simulink model "is95fwdchendtoend2"  (Simulink 4.00)
settings: Solver=VariableStepDiscrete  SolverMode=SingleTasking  StartTime=0.0  StopTime=600  RelTol=1e-3  AbsTol=1e-6
undefined symbols (not defined in the file): Fs
libraries: cdmalibv1p1 x14, cdmaprivate x9, dspsnks3 x3, dspbuff3 x3, commutil2 x3, commsink2 x2, dspsigattribs x2, commchan2 x2
settings Model: RequirementInfo=9  CovMetricSettings=d  Creator=pc  LastModifiedBy=akansal  SaveTime=off  SaveOutput=off  LimitDataPoints=off  ExtModeTrigMode=oneshot  ExtModeArmWhenConnect=off  BlockReductionOpt=off

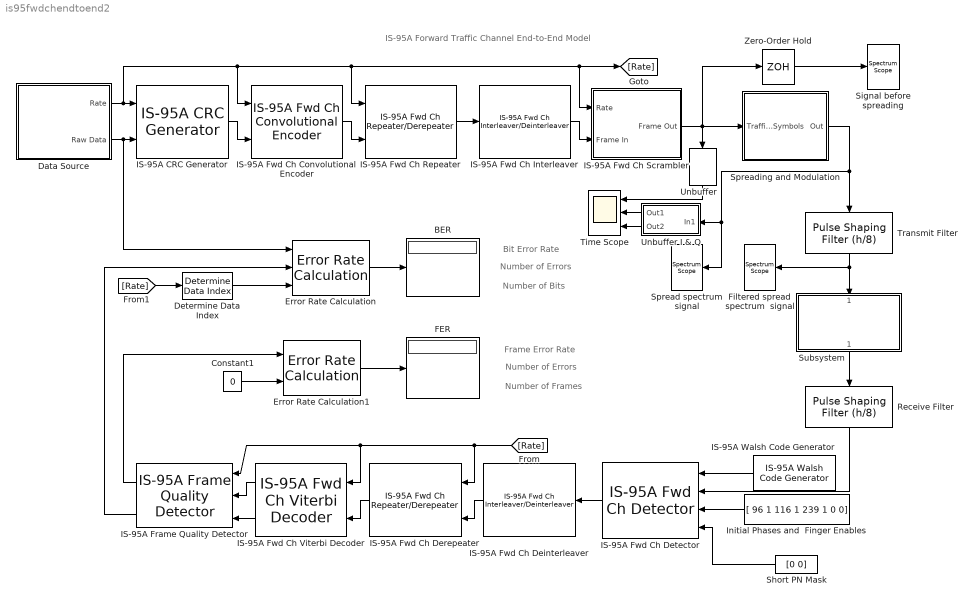
== system is95fwdchendtoend2 ==
  note: IS-95A Forward Traffic Channel
      | End-to-End Model
  note: Frame Error Rate
  note: Number of Errors
  note: Number of Frames
  note: Bit Error Rate
  note: Number of Errors
  note: Number of Bits
  BER : Display
      settings: Format=short
  Constant1 : Constant  Value=0
  Data Source : Subsystem
      settings: RTWFcnNameOpts=Auto  RTWFileNameOpts=Auto
  Determine Data Index : cdmaprivate/Determine Data Index  rateSet=Rate Set I
  Error Rate Calculation : commsink2/Error Rate Calculation  N=2*268  st_delay=2*268  cp_mode=Select samples from port  subframe=[]  PMode=Port  WsName=ErrorVec  RsMode2=off
  Error Rate Calculation1 : commsink2/Error Rate Calculation  N=0  st_delay=4  cp_mode=Entire frame  subframe=[]  PMode=Port  WsName=ErrorVec  RsMode2=off
  FER : Display
      settings: Format=short
  Filtered spread spectrum  signal : dspsnks3/Spectrum Scope  Orientation=left  ScopeProperties=on  Domain=Frequency  HorizSpan=1  UseBuffer=on  BufferSize=8192  Overlap=0  inpFftLenInherit=off  FFTlength=1024  numAvg=10  DisplayProperties=off  AxisGrid=on  Memory=off  FrameNumber=off  AxisLegend=off  AxisZoom=on  OpenScopeAtSimStart=on  OpenScopeImmediately=off  FigPos=[339 281 602 134]  AxisProperties=off  XUnits=Hertz  XRange=[-Fs/2...Fs/2]  InheritXIncr=on  XIncr=1.0  XLabel=Samples  YUnits=dB  YLabel=Magnitude, dB  LineProperties=off
      settings: YMin=-50  YMax=30
  IS-95A CRC Generator : cdmalibv1p1/IS-95A Common/IS-95A CRC Generator  rate_set=Rate Set I  ch_type=Traffic
  IS-95A Frame Quality Detector : cdmalibv1p1/IS-95A Common/IS-95A Frame Quality  Detector  Orientation=left  rateSet=Rate Set I  chType=Traffic  rate2_metric=0.9*1.5  rate3_metric=0.85*1.5
  IS-95A Fwd Ch Convolutional Encoder : cdmalibv1p1/IS-95A Base Station Transmitter/IS-95A Fwd Ch Convolutional Encoder  rate_set=Rate Set I  ch_type=Traffic  enc_state=[]
  IS-95A Fwd Ch Deinterleaver : cdmalibv1p1/IS-95A Base Station Transmitter/IS-95A Fwd Ch Interleaver//Deinterleaver  Orientation=left  ch_type=Traffic  int_select=Deinterleaver
  IS-95A Fwd Ch Derepeater : cdmalibv1p1/IS-95A Base Station Transmitter/IS-95A Fwd Ch Repeater//Derepeater  Orientation=left  rate_set=Rate Set I  ch_type=Traffic  rep_select=Derepeater
  IS-95A Fwd Ch Interleaver : cdmalibv1p1/IS-95A Base Station Transmitter/IS-95A Fwd Ch Interleaver//Deinterleaver  ch_type=Traffic  int_select=Interleaver
  IS-95A Fwd Ch Repeater : cdmalibv1p1/IS-95A Base Station Transmitter/IS-95A Fwd Ch Repeater//Derepeater  rate_set=Rate Set I  ch_type=Traffic  rep_select=Repeater
  IS-95A Fwd Ch Scrambler : Subsystem  mask(IS-95A Fwd Ch Scrambler){rate_set=Rate Set I, chType=Traffic}
      mask prompts: rate_set "Rate Set"; chType "Channel Type"
      mask help: Performs scrambling of the Forward Traffic channel data by the long code and the insertion of power bits in the data.
      settings: RTWFcnNameOpts=Auto  RTWFileNameOpts=Auto
      mask Help: web(cdmaweb);
      mask StyleString: popup(Rate Set I|Rate Set II),popup(Sync|Paging|Traffic)
  IS-95A Fwd Ch Viterbi Decoder : cdmalibv1p1/IS-95A Mobile Station Receiver/IS-95A Fwd Ch Viterbi Decoder  Orientation=left  rateSet=Rate Set I  chType=Traffic  traceBackLenRatio=1  decodeLenRatio=1
  IS-95A Fwd Ch Detector : cdmalibv1p1/IS-95A Mobile Station Receiver/IS-95A Fwd Ch Detector  Orientation=left  rateSet=Rate Set I  numSymb=1  wlshOrd=6  rake_buff_size=3  rake_oversamp=8  sampTime=1/(50*384)
  IS-95A Walsh Code Generator : cdmalibv1p1/IS-95A Common/IS-95A Walsh Code Generator  Orientation=left  wlshOrd=6  wlshIndices=38  st=1/(50*384)
  Initial Phases and  Finger Enables : Constant  Orientation=left  Value=[ 96 1 116 1 239 1 0 0]
  Receive Filter : cdmaprivate/Pulse Shaping Filter (h//8)  Orientation=down  N=1
  Short PN Mask : Constant  Orientation=left  Value=[0 0]
  Signal before spreading : dspsnks3/Spectrum Scope  ScopeProperties=on  Domain=Frequency  HorizSpan=1  UseBuffer=on  BufferSize=1024  Overlap=0  inpFftLenInherit=off  FFTlength=1024  numAvg=10  DisplayProperties=off  AxisGrid=on  Memory=off  FrameNumber=off  AxisLegend=off  AxisZoom=on  OpenScopeAtSimStart=on  OpenScopeImmediately=off  FigPos=[339 599 602 134]  AxisProperties=off  XUnits=Hertz  XRange=[-Fs/2...Fs/2]  InheritXIncr=on  XIncr=1.0  XLabel=Samples  YUnits=dB  YLabel=Magnitude, dB  LineProperties=off
      settings: YMin=-50  YMax=30
  Spread spectrum signal : dspsnks3/Spectrum Scope  Orientation=left  ScopeProperties=on  Domain=Frequency  HorizSpan=1  UseBuffer=on  BufferSize=1024  Overlap=0  inpFftLenInherit=off  FFTlength=1024  numAvg=10  DisplayProperties=off  AxisGrid=on  Memory=off  FrameNumber=off  AxisLegend=off  AxisZoom=on  OpenScopeAtSimStart=on  OpenScopeImmediately=off  FigPos=[339 439 602 134]  AxisProperties=off  XUnits=Hertz  XRange=[-Fs/2...Fs/2]  InheritXIncr=on  XIncr=1.0  XLabel=Samples  YUnits=dB  YLabel=Magnitude, dB  LineProperties=off
      settings: YMin=-50  YMax=30
  Spreading and Modulation : Subsystem
      settings: RTWFcnNameOpts=Auto  RTWFileNameOpts=Auto
      mask Display: disp('Combine with\nSync & Paging\n---\nSS Modulate')
  Subsystem : Subsystem  Orientation=down
      settings: RTWFcnNameOpts=Auto  RTWFileNameOpts=Auto
      mask Display: disp('Rayleigh Multipath\n and  AWGN\nChannel')
  Time Scope : Scope  NumInputPorts=3
      settings: TimeRange=0.001041666666666667  YMin=-3~-3~-3  YMax=3~3~3  SaveToWorkspace=off  SaveName=ScopeData  DataFormat=Structure  LimitDataPoints=on  MaxDataPoints=5000
  Transmit Filter : cdmaprivate/Pulse Shaping Filter (h//8)  Orientation=down  N=8
  Unbuffer : dspbuff3/Unbuffer  Orientation=down  ic=0
  Unbuffer I & Q : Subsystem  Orientation=left
      settings: RTWFcnNameOpts=Auto  RTWFileNameOpts=Auto
      mask Display: disp('Unbuffer\nI & Q');
  Zero-Order Hold : ZeroOrderHold  SampleTime=1/50/384/64
  wires:
  Error Rate Calculation/1 -> BER/1
  [Rate] -> Determine Data Index/1
  Error Rate Calculation1/1 -> FER/1
  Constant1/1 -> Error Rate Calculation1/2
  Determine Data Index/1 -> Error Rate Calculation/3
  Subsystem/1("  ") -> Receive Filter/1
  Initial Phases and  Finger Enables/1 -> IS-95A Fwd Ch Detector/3
  Short PN Mask/1 -> IS-95A Fwd Ch Detector/4
  IS-95A Fwd Ch Deinterleaver/1 -> IS-95A Fwd Ch Derepeater/2
  IS-95A Fwd Ch Derepeater/1 -> IS-95A Fwd Ch Viterbi Decoder/2
  IS-95A Fwd Ch Viterbi Decoder/1 -> IS-95A Frame Quality Detector/2
  IS-95A Fwd Ch Viterbi Decoder/2 -> IS-95A Frame Quality Detector/3
  IS-95A Fwd Ch Detector/1 -> IS-95A Fwd Ch Deinterleaver/1
  Receive Filter/1 -> IS-95A Fwd Ch Detector/2
  IS-95A Frame Quality Detector/1 -> Error Rate Calculation1/1
  IS-95A Frame Quality Detector/2 -> Error Rate Calculation/2
  [Rate] -> IS-95A Fwd Ch Derepeater/1, IS-95A Frame Quality Detector/1, IS-95A Fwd Ch Viterbi Decoder/1
  IS-95A Fwd Ch Repeater/1 -> IS-95A Fwd Ch Interleaver/1
  IS-95A Fwd Ch Convolutional Encoder/1 -> IS-95A Fwd Ch Repeater/2
  Data Source/1(Rate) -> IS-95A Fwd Ch Convolutional Encoder/1, IS-95A Fwd Ch Repeater/1, [Rate], IS-95A Fwd Ch Scrambler/1(Rate), IS-95A CRC Generator/1
  IS-95A Fwd Ch Interleaver/1 -> IS-95A Fwd Ch Scrambler/2(Frame In)
  IS-95A CRC Generator/1 -> IS-95A Fwd Ch Convolutional Encoder/2
  Data Source/2(Raw Data) -> IS-95A CRC Generator/2, Error Rate Calculation/1
  Spreading and Modulation/1("Out ") -> Transmit Filter/1, Unbuffer I & Q/1(In1), Spread spectrum signal/1
  Transmit Filter/1 -> Subsystem/1(" "), Filtered spread spectrum  signal/1
  IS-95A Fwd Ch Scrambler/1(" Frame Out") -> Spreading and Modulation/1(Traffic  Symbols), Unbuffer/1, Zero-Order Hold/1
  IS-95A Walsh Code Generator/1 -> IS-95A Fwd Ch Detector/1
  Unbuffer I & Q/1(Out1) -> Time Scope/2
  Unbuffer I & Q/2(Out2) -> Time Scope/3
  Unbuffer/1 -> Time Scope/1
  Zero-Order Hold/1 -> Signal before spreading/1

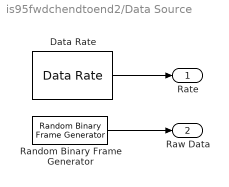
== system is95fwdchendtoend2/Data Source ==
  Data Rate : cdmaprivate/Data Rate  rate=Full
  Random Binary Frame Generator : cdmaprivate/Random Binary Frame Generator  seed=1234  Ts=1/(50*268)  N=268
  Rate : Outport  Port=1  InitialOutput=0
  Raw Data : Outport  Port=2  InitialOutput=0
  wires:
  Data Rate/1 -> Rate/1
  Random Binary Frame Generator/1 -> Raw Data/1

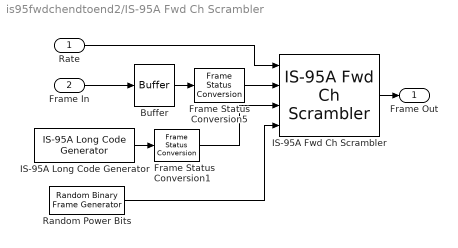
== system is95fwdchendtoend2/IS-95A Fwd Ch Scrambler ==
  Rate : Inport  Port=1  LatchInput=off
  Frame In : Inport  Port=2  LatchInput=off
  Buffer : dspbuff3/Buffer  N=1  V=0  ic=0
  Frame Status Conversion1 : dspsigattribs/Frame Status Conversion  growRefPort=off  outframe=Frame-based
  Frame Status Conversion5 : dspsigattribs/Frame Status Conversion  growRefPort=off  outframe=Frame-based
  IS-95A Fwd Ch Scrambler : cdmalibv1p1/IS-95A Base Station Transmitter/IS-95A Fwd Ch Scrambler  rate_set=Rate Set I  chType=Traffic
  IS-95A Long Code Generator : cdmalibv1p1/IS-95A Common/IS-95A Long Code Generator  num_symb=1  tx_lc_dec_ratio=64  tx_lc_init_mask=2^41  tx_lc_init_state=2^41  tx_sample_time=1/(50*384)
  Random Power Bits : cdmaprivate/Random Binary Frame Generator  seed=956742  Ts=1/50/16  N=1
  " Frame Out" : Outport  Port=1  InitialOutput=0
  wires:
  Rate/1 -> IS-95A Fwd Ch Scrambler/1
  IS-95A Fwd Ch Scrambler/1 -> " Frame Out"/1
  IS-95A Long Code Generator/1 -> Frame Status Conversion1/1
  Frame Status Conversion1/1 -> IS-95A Fwd Ch Scrambler/3
  Random Power Bits/1 -> IS-95A Fwd Ch Scrambler/4
  Buffer/1 -> Frame Status Conversion5/1
  Frame In/1 -> Buffer/1
  Frame Status Conversion5/1 -> IS-95A Fwd Ch Scrambler/2

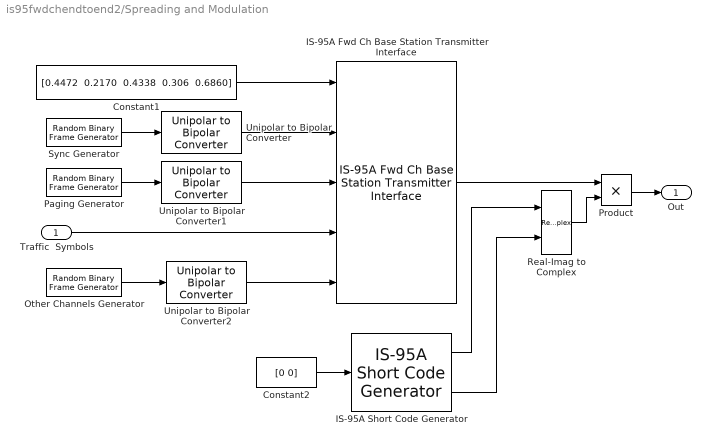
== system is95fwdchendtoend2/Spreading and Modulation ==
  Traffic  Symbols : Inport  Port=1  LatchInput=off
  Constant1 : Constant  Value="[0.4472  0.2170  0.4338  0.306  0.6860]"
  Constant2 : Constant  Value=[0 0]
  IS-95A Fwd Ch Base Station Transmitter Interface : cdmalibv1p1/IS-95A Base Station Transmitter/IS-95A Fwd Ch Base Station Transmitter Interface  paging_rate=Full  wlshOrd=6  wlsh_indices=[0 32 47 38 23]  sampTime=1/(50*384)
  IS-95A Short Code Generator : cdmalibv1p1/IS-95A Common/IS-95A Short Code Generator  numOut=64  sampTime=1/(50*384)
  Other Channels Generator : cdmaprivate/Random Binary Frame Generator  seed=98767657  Ts=1/(50*384)  N=1
  Paging Generator : cdmaprivate/Random Binary Frame Generator  seed=76767  Ts=1/(50*384)  N=1
  Product : Product  Inputs=2  Multiplication=Element-wise(.*)  SaturateOnIntegerOverflow=on
  Real-Imag to Complex : RealImagToComplex  Input=RealAndImag  ConstantPart=0
  Sync Generator : cdmaprivate/Random Binary Frame Generator  seed=465789  Ts=4 * 1/(50*384)  N=1
  Unipolar to Bipolar Converter : commutil2/Unipolar to Bipolar Converter  M=2  polarity=Negative
  Unipolar to Bipolar Converter1 : commutil2/Unipolar to Bipolar Converter  M=2  polarity=Negative
  Unipolar to Bipolar Converter2 : commutil2/Unipolar to Bipolar Converter  M=2  polarity=Negative
  "Out " : Outport  Port=1  InitialOutput=0
  wires:
  Sync Generator/1 -> Unipolar to Bipolar Converter/1
  Paging Generator/1 -> Unipolar to Bipolar Converter1/1
  Other Channels Generator/1 -> Unipolar to Bipolar Converter2/1
  Constant2/1 -> IS-95A Short Code Generator/1
  Constant1/1 -> IS-95A Fwd Ch Base Station Transmitter Interface/1
  Unipolar to Bipolar Converter/1 -> IS-95A Fwd Ch Base Station Transmitter Interface/2
  Unipolar to Bipolar Converter1/1 -> IS-95A Fwd Ch Base Station Transmitter Interface/3
  Traffic  Symbols/1 -> IS-95A Fwd Ch Base Station Transmitter Interface/4
  Unipolar to Bipolar Converter2/1 -> IS-95A Fwd Ch Base Station Transmitter Interface/5
  Real-Imag to Complex/1 -> Product/2
  IS-95A Fwd Ch Base Station Transmitter Interface/1 -> Product/1
  Product/1 -> "Out "/1
  IS-95A Short Code Generator/1 -> Real-Imag to Complex/1
  IS-95A Short Code Generator/2 -> Real-Imag to Complex/2

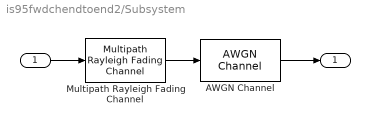
== system is95fwdchendtoend2/Subsystem ==
  " " : Inport  Port=1  LatchInput=off
  AWGN Channel : commchan2/AWGN Channel  seed=17583  noiseMode="Signal to noise ratio  (Es/No)"  EsNodB=-3.0  SNRdB=10  Ps=2  Tsym=1/1228800  variance=1
  Multipath Rayleigh Fading Channel : commchan2/Multipath Rayleigh Fading Channel  Fd=175.92  simTs=1/(1228800*8)  delayVec=[0 2e-6 14.5e-6]  gainVecdB=[0 0 -3]  normGain=on  Seed=1234
  "  " : Outport  Port=1
  wires:
  AWGN Channel/1 -> "  "/1
  " "/1 -> Multipath Rayleigh Fading Channel/1
  Multipath Rayleigh Fading Channel/1 -> AWGN Channel/1

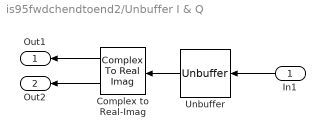
== system is95fwdchendtoend2/Unbuffer I & Q ==
  In1 : Inport  Orientation=left  Port=1  LatchInput=off
  Complex to Real-Imag : ComplexToRealImag  Orientation=left  Output=RealAndImag
  Unbuffer : dspbuff3/Unbuffer  Orientation=left  ic=0
  Out1 : Outport  Orientation=left  Port=1
  Out2 : Outport  Orientation=left  Port=2
  wires:
  Unbuffer/1 -> Complex to Real-Imag/1
  Complex to Real-Imag/1 -> Out1/1
  Complex to Real-Imag/2 -> Out2/1
  In1/1 -> Unbuffer/1
